simulink model "MPC_FOC"  (R2021a)
settings: Solver=VariableStepAuto  StartTime=0.0  StopTime=2  RelTol=1e-3
undefined symbols (not defined in the file): C1, JL, JM, K1, sigbuilder_block
libraries: powerlib_extras x9, spsDCVoltageSourceLib x4, spsPermanentMagnetSynchronousMachineLib x4, spsUniversalBridgeLib x4, spspowerguiLib x4, simulink x3, spsVoltageMeasurementLib x3, pid_lib x1
(part 1 of 2)
settings Model: Creator=86188  LastModifiedBy=86188

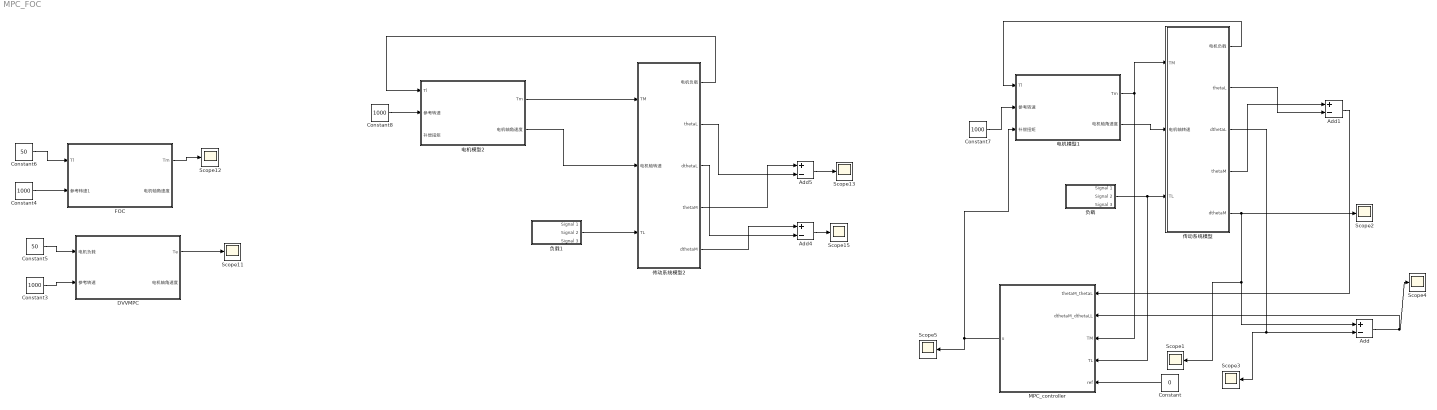
== system MPC_FOC ==
  Add{,1,4..5} (4 alike) : Sum  Inputs=+-
  Constant : Constant  Value=0
  Constant{3..4,7..8} (4 alike) : Constant  Value=1000
  Constant5 : Constant  Value=50
  Constant6 : Constant  Value=50
  DVVMPC : Subsystem
  FOC : Subsystem
  MPC_controller : MATLAB Function  TreatAsAtomicUnit=on
  Scope{1..5,11..13,15} (9 alike) : Scope
  传动系统模型 : Subsystem
  传动系统模型2 : Subsystem
  电机模型1 : Subsystem
  电机模型2 : Subsystem
  负载 : Subsystem  Tag=STV Subsys  LoadFcn=sigbuilder_block('load');  StartFcn=sigbuilder_block('start');  StopFcn=sigbuilder_block('stop');  ClipboardFcn=sigbuilder_block('clipboard');  mask(Sigbuilder block){tuvar=[0:10]}
      mask help: Simulink:masks:SigbuilderBlock_MD
      mask init:
      | if ~strcmp(get_param(bdroot(gcbh),'SimulationStatus'),'stopped') tuvar = sigbuilder_block('maskInit'); end
      settings: CopyFcn=sigbuilder_block('copy');  DeleteFcn=sigbuilder_block('delete');  ModelCloseFcn=sigbuilder_block('modelClose');  PreSaveFcn=sigbuilder_block('preSave');  PauseFcn=sigbuilder_block('pause');  ContinueFcn=sigbuilder_block('continue');  NameChangeFcn=sigbuilder_block('namechange');  OpenFcn=sigbuilder_block('open',[5.4 36 1141.2 517.8 ]);  CloseFcn=sigbuilder_block('close');
      mask Display: plot(0, 0, 100, 100,[2, 2, 32, 32, 2], [68, 8, 8, 68, 68],[32, 2], [38, 38], [32, 19, 2],[53, 60, 44], [32, 17, 17, 2],[16, 16, 31, 31]);txt = getActiveGroup(gcbh);text(2, 100, txt,'verticalAlignment', 'top');
  负载1 : Subsystem  Tag=STV Subsys  LoadFcn=sigbuilder_block('load');  StartFcn=sigbuilder_block('start');  StopFcn=sigbuilder_block('stop');  ClipboardFcn=sigbuilder_block('clipboard');  mask(Sigbuilder block){tuvar=[0:10]}
      mask help: Simulink:masks:SigbuilderBlock_MD
      mask init:
      | if ~strcmp(get_param(bdroot(gcbh),'SimulationStatus'),'stopped') tuvar = sigbuilder_block('maskInit'); end
      settings: CopyFcn=sigbuilder_block('copy');  DeleteFcn=sigbuilder_block('delete');  ModelCloseFcn=sigbuilder_block('modelClose');  PreSaveFcn=sigbuilder_block('preSave');  PauseFcn=sigbuilder_block('pause');  ContinueFcn=sigbuilder_block('continue');  NameChangeFcn=sigbuilder_block('namechange');  OpenFcn=sigbuilder_block('open',[5.4 36 1141.2 517.8 ]);  CloseFcn=sigbuilder_block('close');
      mask Display: plot(0, 0, 100, 100,[2, 2, 32, 32, 2], [68, 8, 8, 68, 68],[32, 2], [38, 38], [32, 19, 2],[53, 60, 44], [32, 17, 17, 2],[16, 16, 31, 31]);txt = getActiveGroup(gcbh);text(2, 100, txt,'verticalAlignment', 'top');
  wires:
  传动系统模型/1(电机负载) -> 电机模型1/1(Tl)
  传动系统模型/3(dthetaL) -> Scope3/1, Add/2
  负载/2(Signal 2) -> MPC_controller/4(TL), 传动系统模型/3(TL)
  Add/1 -> MPC_controller/2(dthetaM_dthetaLL), Scope4/1
  传动系统模型/5(dthetaM) -> Scope2/1, Add/1, Scope1/1
  电机模型1/2(电机轴角速度) -> 传动系统模型/2(电机轴转速)
  传动系统模型/2(thetaL) -> Add1/2
  传动系统模型/4(thetaM) -> Add1/1
  Add1/1 -> MPC_controller/1(thetaM_thetaL)
  Constant/1 -> MPC_controller/5(ref)
  MPC_controller/1(u) -> Scope5/1, 电机模型1/3(补偿扭矩)
  电机模型1/1(Tm) -> MPC_controller/3(TM), 传动系统模型/1(TM)
  Constant7/1 -> 电机模型1/2(参考转速)
  Constant3/1 -> DVVMPC/2(参考转速)
  Constant5/1 -> DVVMPC/1(电机负载)
  Constant6/1 -> FOC/1(Tl)
  DVVMPC/1(Te) -> Scope11/1
  FOC/1(Tm) -> Scope12/1
  传动系统模型2/4(thetaM) -> Add5/1
  传动系统模型2/1(电机负载) -> 电机模型2/1(Tl)
  电机模型2/2(电机轴角速度) -> 传动系统模型2/2(电机轴转速)
  传动系统模型2/2(thetaL) -> Add5/2
  电机模型2/1(Tm) -> 传动系统模型2/1(TM)
  Constant8/1 -> 电机模型2/2(参考转速)
  负载1/2(Signal 2) -> 传动系统模型2/3(TL)
  Constant4/1 -> FOC/2(参考转速1)
  Add5/1 -> Scope13/1
  Add4/1 -> Scope15/1
  传动系统模型2/5(dthetaM) -> Add4/1
  传动系统模型2/3(dthetaL) -> Add4/2

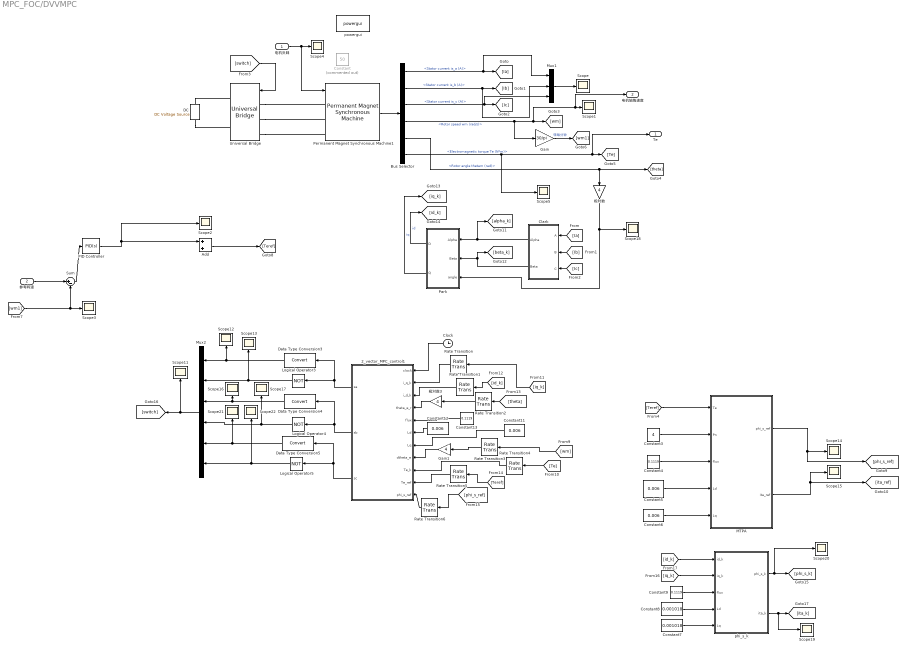
== system MPC_FOC/DVVMPC ==
  电机负载 : Inport
  参考转速 : Inport  Port=2
  2_vector_MPC_control1 : MATLAB Function  TreatAsAtomicUnit=on  SystemSampleTime=1e-5
  Add : Sum
  Bus Selector : BusSelector  OutputSignals=Stator current is_a (A),Stator current is_b (A),Stator current is_c (A),Rotor speed wm (rad/s),Rotor angle thetam (rad),Electromagnetic torque Te (N*m)
  Clark : Subsystem
  Clock : Clock
  Constant : Constant  Commented=on  Value=50
  Constant{5..6,11..12} (4 alike) : Constant  Value=0.006
  Constant13 : Constant  Value=0.1119
  Constant3 : Constant  Value=4
  Constant4 : Constant  Value=0.1119
  Constant7 : Constant  Value=0.001018
  Constant8 : Constant  Value=0.001018
  Constant9 : Constant  Value=0.1119
  DC : spsDCVoltageSourceLib/DC Voltage Source  Amplitude=400  Measurements=None
  Data Type Conversion3 : DataTypeConversion
  Data Type Conversion4 : DataTypeConversion
  Data Type Conversion5 : DataTypeConversion
  Gain : Gain  Gain=30/pi
  Gain1 : Gain  Gain=4
  Logical Operator3 : Logic  Operator=NOT  AllPortsSameDT=off  OutDataTypeStr=boolean
  Logical Operator4 : Logic  Operator=NOT  AllPortsSameDT=off  OutDataTypeStr=boolean
  Logical Operator5 : Logic  Operator=NOT  AllPortsSameDT=off  OutDataTypeStr=boolean
  MTPA : MATLAB Function  TreatAsAtomicUnit=on
  Mux1 : Mux  Inputs=3
  Mux2 : Mux  Inputs=6
  PID Controller : pid_lib/PID Controller  Controller=PID  Form=Parallel  TimeDomain=Continuous-time  UseExternalTs=off  SampleTime=-1  IntegratorMethod=Forward Euler  FilterMethod=Forward Euler  ControllerParametersSource=internal  P=2  I=0.125  D=0.01  UseFilter=on  N=100  TunerSelectOption=Transfer Function Based (PID Tuner App)  InitialConditionSource=internal  InitialConditionForIntegrator=0  InitialConditionForFilter=0  DifferentiatorICPrevScaledInput=0  ExternalReset=none  TrackingMode=off  Kt=1  LimitOutput=on  SatLimitsSource=internal  UpperSaturationLimit=140  LowerSaturationLimit=-200  LinearizeAsGain=on  AntiWindupMode=none  Kb=1  POutMin=[]  POutMax=[]  IOutMin=[]  IOutMax=[]  DOutMin=[]  DOutMax=[]  NOutMin=[]  NOutMax=[]  SumOutMin=[]  SumOutMax=[]  SaturationOutMin=[]  SaturationOutMax=[]  PParamMin=[]  PParamMax=[]  IParamMin=[]  IParamMax=[]  DParamMin=[]  DParamMax=[]  NParamMin=[]  NParamMax=[]  KbParamMin=[]  KbParamMax=[]  KtParamMin=[]  KtParamMax=[]  KbOutMin=[]  KbOutMax=[]  KtOutMin=[]  KtOutMax=[]  IntegratorOutMin=[]  IntegratorOutMax=[]  FilterOutMin=[]  FilterOutMax=[]  SumI1OutMin=[]  SumI1OutMax=[]  SumI2OutMin=[]  SumI2OutMax=[]  SumI3OutMin=[]  SumI3OutMax=[]  SumI4OutMin=[]  SumI4OutMax=[]  SumDOutMin=[]  SumDOutMax=[]  DifferentiatorOutMin=[]  DifferentiatorOutMax=[]  FilterDiffOutCoefMin=[]  FilterDiffOutCoefMax=[]  ReciprocalOutMin=[]  ReciprocalOutMax=[]  SumDenOutMin=[]  SumDenOutMax=[]  SumNumOutMin=[]  SumNumOutMax=[]  DivideOutMin=[]  DivideOutMax=[]  UdiffTsProdOutMin=[]  UdiffTsProdOutMax=[]  NTsProdOutMin=[]  NTsProdOutMax=[]  UintegralTsProdOutMin=[]  UintegralTsProdOutMax=[]  UngainTsProdOutMin=[]  UngainTsProdOutMax=[]  IntegratorContinuousStateAttributes=''  IntegratorStateMustResolveToSignalObject=off  IntegratorRTWStateStorageClass=Auto  FilterContinuousStateAttributes=''  FilterStateMustResolveToSignalObject=off  FilterRTWStateStorageClass=Auto  ParallelPVariant=InternalParameters  IdealPVariant=Disabled  IVariant=InternalParameters  DVariant=InternalParameters  IntegratorVariant=Continuous  SatVariant=Enabled  AWVariant=Passthrough  PCopyVariant=Disabled  TRVariant=Disabled  FdbkBlocksVariant=Forward  IdealPFdbkVariant=Disabled  SatFdbkVariant=Disabled  DerivativeFilterVariant=ContFilter  NVariant=InternalParameters  NCopyVariant=Disabled  FilterICVariant=InternalICsFilter  IntegratorICVariant=InternalICs  ExternalResetVariant=Disabled  TRSumVariant=Passthrough  SumFdbkVariant=Disabled  SumVariant=Sum_PID  TsampFilterVariant=InternalTs  TsampNgainVariant=Passthrough  TsampIntegralVariant=Passthrough  ExternalSaturationOutDataTypeStr=Inherit: Same as second input
  Park : Subsystem
  Permanent Magnet Synchronous Machine1 : spsPermanentMagnetSynchronousMachineLib/Permanent Magnet Synchronous Machine  NbPhases=3  FluxDistribution=Sinusoidal  RotorType=Salient-pole  MechanicalLoad=Torque Tm  PresetModel=No  ShowDetailedParameters=on  MeasurementBus=off  Resistance=0.11  Inductance=8.5e-3  dqInductances=[0.006 0.006]  La=0.000835  MachineConstant=Flux linkage established by magnets (V.s)  Flux=0.1119  VoltageCst=81.1857  TorqueCst=0.6714  Flat=120  Mechanical=[0.04 0.0002024 4 0]  PolePairs=4  InitialConditions=[0,0, 0,0]  InitialConditions5ph=[0 0 0 0 0 0]  RefAngle=Aligned with phase A axis (original Park)  IterativeDiscreteModel=Trapezoidal non iterative  TsBlock=-1  TsPowergui=0
  Rate Transition{,1..6} (7 alike) : RateTransition  OutPortSampleTime=1e-4
  Scope{,1..5,11..22} (18 alike) : Scope
  Sum : Sum  Inputs=|+-
  Universal Bridge : spsUniversalBridgeLib/Universal Bridge  Arms=3  SnubberResistance=1e5  SnubberCapacitance=inf  Device=IGBT / Diodes  Ron=1e-3  Lon=0  ForwardVoltages="[  0  0  ]"  ForwardVoltage=0  GTOparameters=[ 10e-6 , 20e-6 ]  IGBTparameters=[ 1e-6 , 2e-6 ]  Measurements=None  Measurements_2=None  converterType=Rectifier
  phi_s_k : MATLAB Function  TreatAsAtomicUnit=on
  powergui : spspowerguiLib/powergui  Priority=1  SimulationMode=Discrete  SampleTime=1e-6  frequency=60  Iterations=50  frequencyindice=0  Pbase=100e6  ErrMax=1e-4  UnitsV=kV  UnitsW=MW  buscounter=0  FunctionMessages=off  echomessages=off  EnableUseOfTLC=off  CurrentSourceSwitches=off  DisableSnubberDevices=off  DisableRonSwitches=off  DisableVfSwitches=off  DisplayEquations=off  AutomaticDiscreteSolvers=off  SolverType=Tustin/Backward Euler (TBE)  Interpol=off  ExternalGateDelay=off  methode=off  Ts=100  x0status=blocks  SPID=on  SwTol=0  HookPort=off  NonlinearTolerance=1e-4  nMaxIteration=100  ContinueOnMaxIteration=off  RestoreLinks=warning  ResistiveCurrentMeasurement=off  Frange=[0:2:500]  Ylog=off  Xlog=on  ShowGrid=off  save=off  variable=ZData  structure=0  ZoomFFT=off  StartTime=0.0  cycles=1  DisplayStyle=1  fundamental=60  FreqAxis=off  MaxFrequency=1000  frequencyindicesteady=1  RmsSteady=1  display=off
  极对数 : Gain  Gain=4
  极对数3 : Gain  Gain=4
  Te : Outport
  电机轴角速度 : Outport  Port=2
  wires:
  参考转速/1 -> Sum/1
  Add/1 -> [Teref]
  电机负载/1 -> Scope4/1, Permanent Magnet Synchronous Machine1/1
  Rate Transition6/1 -> 2_vector_MPC_control1/11(phi_s_ref)
  Rate Transition5/1 -> 2_vector_MPC_control1/10(Te_ref)
  Rate Transition4/1 -> 2_vector_MPC_control1/9(Te_k)
  Rate Transition3/1 -> Gain1/1
  Rate Transition2/1 -> 极对数3/1
  Rate Transition1/1 -> 2_vector_MPC_control1/3(i_d_k)
  Rate Transition/1 -> 2_vector_MPC_control1/2(i_q_k)
  phi_s_k/2(ita_k) -> [ita_k], Scope19/1
  极对数3/1 -> 2_vector_MPC_control1/4(theta_e_r)
  Mux2/1 -> [switch], Scope11/1
  Logical Operator5/1 -> Scope22/1, Mux2/6
  Data Type Conversion5/1 -> Scope21/1, Mux2/5
  Logical Operator4/1 -> Scope17/1, Mux2/4
  Data Type Conversion4/1 -> Scope16/1, Mux2/3
  Logical Operator3/1 -> Scope13/1, Mux2/2
  Data Type Conversion3/1 -> Scope12/1, Mux2/1
  2_vector_MPC_control1/3(sc) -> Logical Operator5/1, Data Type Conversion5/1
  2_vector_MPC_control1/2(sb) -> Logical Operator4/1, Data Type Conversion4/1
  2_vector_MPC_control1/1(sa) -> Logical Operator3/1, Data Type Conversion3/1
  [id_k] -> phi_s_k/1(id_k)
  [iq_k] -> phi_s_k/2(iq_k)
  phi_s_k/1(phi_s_k) -> Scope20/1, [phi_s_k]
  Constant9/1 -> phi_s_k/3(flux)
  Constant8/1 -> phi_s_k/4(Ld)
  Constant7/1 -> phi_s_k/5(Lq)
  MTPA/1(phi_s_ref) -> Scope14/1, [phi_s_ref]
  MTPA/2(ita_ref) -> [ita_ref], Scope15/1
  Constant6/1 -> MTPA/5(Lq)
  Constant5/1 -> MTPA/4(Ld)
  Constant4/1 -> MTPA/3(flux)
  Constant3/1 -> MTPA/2(Pn)
  [Teref] -> MTPA/1(Te)
  Clock/1 -> 2_vector_MPC_control1/1(clock)
  Permanent Magnet Synchronous Machine1/1 -> Bus Selector/1
  Bus Selector/1 -> Mux1/1, [Ia]  "<Stator current is_a (A)>"
  Bus Selector/2 -> Mux1/2, [Ib]  "<Stator current is_b (A)>"
  Bus Selector/3 -> Mux1/3, [Ic]  "<Stator current is_c (A)>"
  Bus Selector/4 -> Gain/1, Scope1/1, 电机轴角速度/1, [wm]  "<Rotor speed wm (rad/s)>"
  Bus Selector/5 -> 极对数/1, [theta]  "<Rotor angle thetam (rad)>"
  Bus Selector/6 -> [Te], Te/1, Scope5/1  "<Electromagnetic torque Te (N*m)>"
  Gain/1 -> [wm1]  "转每分钟"
  Clark/1(Alpha) -> Park/1(Alpha), [alpha_k]
  Clark/2(Beta) -> Park/2(Beta), [beta_k]
  [Ia] -> Clark/1(A)
  [Ib] -> Clark/2(B)
  [Ic] -> Clark/3(C)
  极对数/1 -> Park/3(angle), Scope18/1
  Park/1(D) -> [id_k]  "id"
  Park/2(Q) -> [iq_k]  "iq"
  [switch] -> Universal Bridge/1
  Mux1/1 -> Scope/1
  Sum/1 -> PID Controller/1
  [wm1] -> Scope3/1, Sum/2
  PID Controller/1 -> Scope2/1, Add/1
  Gain1/1 -> 2_vector_MPC_control1/8(dtheta_e)
  Constant12/1 -> 2_vector_MPC_control1/6(Ld)
  Constant11/1 -> 2_vector_MPC_control1/7(Lq)
  Constant13/1 -> 2_vector_MPC_control1/5(flux)
  [Teref] -> Rate Transition5/1
  [phi_s_ref] -> Rate Transition6/1
  [iq_k] -> Rate Transition/1
  [id_k] -> Rate Transition1/1
  [theta] -> Rate Transition2/1
  [wm] -> Rate Transition3/1
  [Te] -> Rate Transition4/1
  connections:
  Universal Bridge/LConn2 -- Permanent Magnet Synchronous Machine1/LConn2
  Universal Bridge/LConn3 -- Permanent Magnet Synchronous Machine1/LConn3
  Universal Bridge/LConn1 -- Permanent Magnet Synchronous Machine1/LConn1
  DC/RConn1 -- Universal Bridge/RConn1
  DC/LConn1 -- Universal Bridge/RConn2

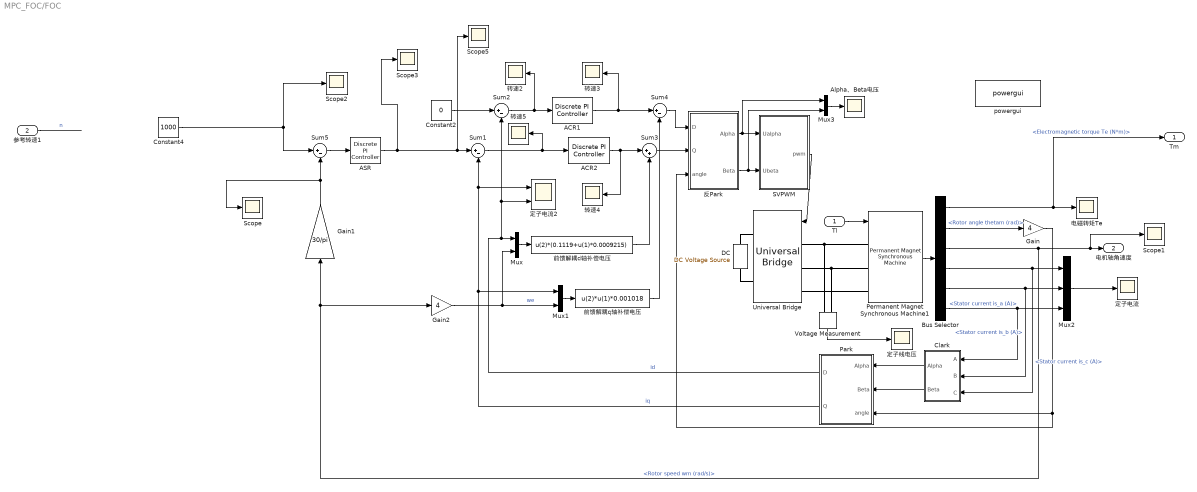
== system MPC_FOC/FOC ==
  Tl : Inport
  参考转速1 : Inport  Port=2
  ACR1 : powerlib_extras/Discrete  Control Blocks/Discrete PI Controller  Kp=4  Ki=80  Par_Limits=[560*0.9*sqrt(1/3) -560*0.9*sqrt(1/3)]  Init=0  Ts=1e-6
  ACR2 : powerlib_extras/Discrete  Control Blocks/Discrete PI Controller  Kp=4  Ki=80  Par_Limits=[560*0.9*sqrt(1/3) -560*0.9*sqrt(1/3)]  Init=0  Ts=1e-6
  ASR : powerlib_extras/Discrete  Control Blocks/Discrete PI Controller  Kp=5  Ki=200  Par_Limits=[200 -200]  Init=0  Ts=1e-6
  Alpha、Beta电压 : Scope
  Bus Selector : BusSelector  OutputSignals=Electromagnetic torque Te (N*m),Rotor angle thetam (rad),Rotor speed wm (rad/s),Stator current is_c (A),Stator current is_b (A),Stator current is_a (A)
  Clark : Subsystem
  Constant2 : Constant  Value=0
  Constant4 : Constant  Value=1000
  DC : spsDCVoltageSourceLib/DC Voltage Source  Amplitude=560  Measurements=None
  Gain : Gain  Gain=4
  Gain1 : Gain  Gain=30/pi
  Gain2 : Gain  Gain=4
  Mux : Mux  Inputs=2
  Mux1 : Mux  Inputs=2
  Mux2 : Mux  Inputs=3
  Mux3 : Mux  Inputs=2
  Park : Subsystem
  Permanent Magnet Synchronous Machine1 : spsPermanentMagnetSynchronousMachineLib/Permanent Magnet Synchronous Machine  NbPhases=3  FluxDistribution=Sinusoidal  RotorType=Salient-pole  MechanicalLoad=Torque Tm  PresetModel=No  ShowDetailedParameters=on  MeasurementBus=off  Resistance=0.11  Inductance=8.5e-3  dqInductances=[0.0009215 0.001018]  La=0.000835  MachineConstant=Flux linkage established by magnets (V.s)  Flux=0.1119  VoltageCst=81.1857  TorqueCst=0.6714  Flat=120  Mechanical=[0.04 0.0002024 4 0]  PolePairs=4  InitialConditions=[0,0, 0,0]  InitialConditions5ph=[0 0 0 0 0 0]  RefAngle=Aligned with phase A axis (original Park)  IterativeDiscreteModel=Trapezoidal non iterative  TsBlock=-1  TsPowergui=0
  SVPWM : Subsystem
  Scope{,1..3,5} (5 alike) : Scope
  Sum{1..2,4..5} (4 alike) : Sum  Inputs=|+-
  Sum3 : Sum  Inputs=|++
  Universal Bridge : spsUniversalBridgeLib/Universal Bridge  Arms=3  SnubberResistance=1e5  SnubberCapacitance=inf  Device=IGBT / Diodes  Ron=1e-3  Lon=0  ForwardVoltages="[  0  0  ]"  ForwardVoltage=0  GTOparameters=[ 10e-6 , 20e-6 ]  IGBTparameters=[ 1e-6 , 2e-6 ]  Measurements=None  Measurements_2=None  converterType=Rectifier
  Voltage Measurement : spsVoltageMeasurementLib/Voltage Measurement  PhasorSimulation=off  OutputType=Complex  PSBequivalent=0
  powergui : spspowerguiLib/powergui  Priority=1  SimulationMode=Discrete  SampleTime=1e-5  frequency=60  Iterations=50  frequencyindice=0  Pbase=100e6  ErrMax=1e-4  UnitsV=kV  UnitsW=MW  buscounter=0  FunctionMessages=off  echomessages=off  EnableUseOfTLC=off  CurrentSourceSwitches=off  DisableSnubberDevices=off  DisableRonSwitches=off  DisableVfSwitches=off  DisplayEquations=off  AutomaticDiscreteSolvers=off  SolverType=Tustin  Interpol=off  ExternalGateDelay=off  methode=off  Ts=0  x0status=blocks  SPID=off  SwTol=0  HookPort=off  NonlinearTolerance=1e-4  nMaxIteration=100  ContinueOnMaxIteration=off  RestoreLinks=warning  ResistiveCurrentMeasurement=off  Frange=[0:2:500]  Ylog=off  Xlog=on  ShowGrid=off  save=off  variable=ZData  structure=ScopeData7  ZoomFFT=on  StartTime=2.5  cycles=3  DisplayStyle=1  fundamental=60  FreqAxis=off  MaxFrequency=2000  frequencyindicesteady=1  RmsSteady=1  display=off
  前馈解耦d轴补偿电压 : Fcn  Expr=u(2)*(0.1119+u(1)*0.0009215)
  前馈解耦q轴补偿电压 : Fcn  Expr=u(2)*u(1)*0.001018
  反Park : Subsystem
  定子电流 : Scope
  定子电流2 : Scope  NumInputPorts=2
  定子线电压 : Scope
  电磁转矩Te : Scope
  转速{2..5} (4 alike) : Scope
  Tm : Outport
  电机轴角速度 : Outport  Port=2
  wires:
  ASR/1 -> Sum1/1, Scope5/1, Scope3/1
  Constant4/1 -> Scope2/1, Sum5/1
  Gain1/1 -> Scope/1, Sum5/2
  Tl/1 -> Permanent Magnet Synchronous Machine1/1
  Voltage Measurement/1 -> 定子线电压/1
  前馈解耦q轴补偿电压/1 -> Sum4/2
  Sum2/1 -> ACR1/1, 转速2/1
  Mux2/1 -> 定子电流/1
  Bus Selector/6 -> Clark/1(A), Mux2/3  "<Stator current is_a (A)>"
  Sum5/1 -> ASR/1
  Clark/1(Alpha) -> Park/1(Alpha)
  Permanent Magnet Synchronous Machine1/1 -> Bus Selector/1
  Park/2(Q) -> Sum1/2, 定子电流2/1, Mux1/1  "iq"
  Clark/2(Beta) -> Park/2(Beta)
  Sum1/1 -> ACR2/1, 转速5/1
  Mux3/1 -> Alpha、Beta电压/1
  反Park/1(Alpha) -> SVPWM/1(Ualpha), Mux3/1
  Bus Selector/3 -> 电机轴角速度/1, Scope1/1, Gain1/1, Gain2/1  "<Rotor speed wm (rad/s)>"
  Mux/1 -> 前馈解耦d轴补偿电压/1
  反Park/2(Beta) -> SVPWM/2(Ubeta), Mux3/2
  Sum3/1 -> 反Park/2(Q)
  Park/1(D) -> Mux/1, Sum2/2, 定子电流2/2  "id"
  Bus Selector/1 -> 电磁转矩Te/1, Tm/1  "<Electromagnetic torque Te (N*m)>"
  Bus Selector/5 -> Clark/2(B), Mux2/2  "<Stator current is_b (A)>"
  Bus Selector/2 -> Gain/1  "<Rotor angle thetam (rad)>"
  前馈解耦d轴补偿电压/1 -> Sum3/2
  ACR2/1 -> Sum3/1, 转速4/1
  Sum4/1 -> 反Park/1(D)
  SVPWM/1(pwm) -> Universal Bridge/1
  Mux1/1 -> 前馈解耦q轴补偿电压/1
  Gain2/1 -> Mux/2, Mux1/2  "we"
  Gain/1 -> Park/3(angle), 反Park/3(angle)
  Constant2/1 -> Sum2/1
  Bus Selector/4 -> Clark/3(C), Mux2/1  "<Stator current is_c (A)>"
  ACR1/1 -> Sum4/1, 转速3/1
  参考转速1/1 -> ?  "n"
  connections:
  Voltage Measurement/LConn1 -- Permanent Magnet Synchronous Machine1/LConn1 -- Universal Bridge/LConn1
  Voltage Measurement/LConn2 -- Permanent Magnet Synchronous Machine1/LConn2 -- Universal Bridge/LConn2
  DC/RConn1 -- Universal Bridge/RConn1
  Permanent Magnet Synchronous Machine1/LConn3 -- Universal Bridge/LConn3
  DC/LConn1 -- Universal Bridge/RConn2

== system MPC_FOC/传动系统模型 ==
  TM : Inport
  电机轴转速 : Inport  Port=2
  TL : Inport  Port=3
  Fcn1 : Subsystem
  Fcn2 : Subsystem
  电机负载 : Outport
  thetaL : Outport  Port=2
  dthetaL : Outport  Port=3
  thetaM : Outport  Port=4
  dthetaM : Outport  Port=5
  wires:
  Fcn2/1(d2thetaL) -> Fcn1/2(d2theta1)
  TM/1 -> Fcn1/1(TM)
  电机轴转速/1 -> Fcn1/3(电机轴转速)
  Fcn1/1(d2theta) -> Fcn2/2(d2thata)
  Fcn1/2(电机负载) -> 电机负载/1
  Fcn1/3(thetaM) -> thetaM/1
  Fcn1/4(dthetaM) -> dthetaM/1
  TL/1 -> Fcn2/1(TL)
  Fcn2/2(thetaL) -> thetaL/1
  Fcn2/3(dthetaL) -> dthetaL/1

== system MPC_FOC/传动系统模型2 ==
  TM : Inport
  电机轴转速 : Inport  Port=2
  TL : Inport  Port=3
  Fcn1 : Subsystem
  Fcn2 : Subsystem
  电机负载 : Outport
  thetaL : Outport  Port=2
  dthetaL : Outport  Port=3
  thetaM : Outport  Port=4
  dthetaM : Outport  Port=5
  wires:
  Fcn2/3(dthetaL) -> dthetaL/1
  Fcn2/2(thetaL) -> thetaL/1
  TL/1 -> Fcn2/1(TL)
  Fcn1/4(dthetaM) -> dthetaM/1
  Fcn1/3(thetaM) -> thetaM/1
  Fcn1/2(电机负载) -> 电机负载/1
  Fcn1/1(d2theta) -> Fcn2/2(d2thata)
  电机轴转速/1 -> Fcn1/3(电机轴转速)
  TM/1 -> Fcn1/1(TM)
  Fcn2/1(d2thetaL) -> Fcn1/2(d2theta1)

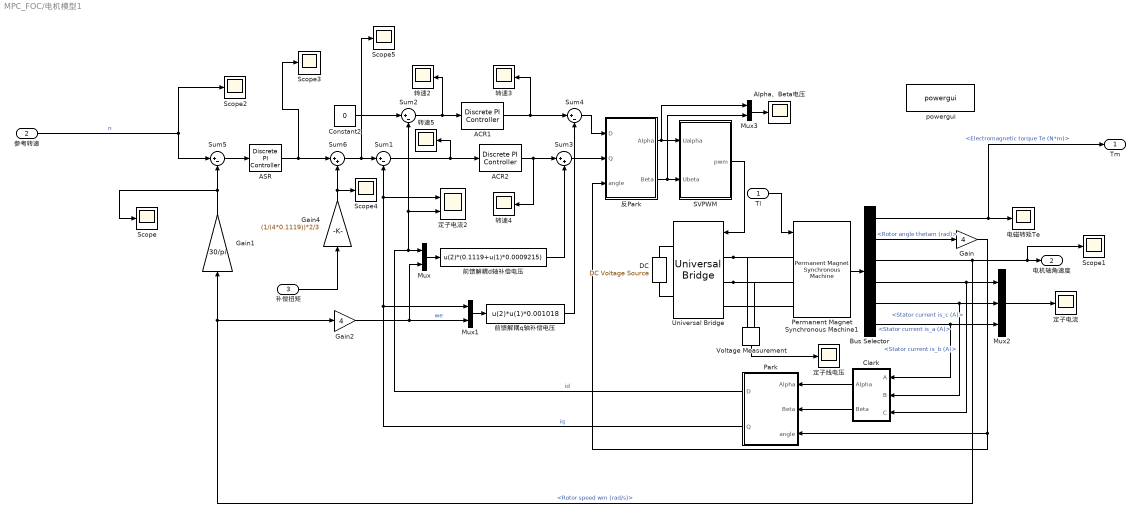
== system MPC_FOC/电机模型1 ==
  Tl : Inport
  参考转速 : Inport  Port=2
  补偿扭矩 : Inport  Port=3
  ACR1 : powerlib_extras/Discrete  Control Blocks/Discrete PI Controller  Kp=4  Ki=80  Par_Limits=[560*0.9*sqrt(1/3) -560*0.9*sqrt(1/3)]  Init=0  Ts=1e-6
  ACR2 : powerlib_extras/Discrete  Control Blocks/Discrete PI Controller  Kp=4  Ki=80  Par_Limits=[560*0.9*sqrt(1/3) -560*0.9*sqrt(1/3)]  Init=0  Ts=1e-6
  ASR : powerlib_extras/Discrete  Control Blocks/Discrete PI Controller  Kp=5  Ki=200  Par_Limits=[200 -200]  Init=0  Ts=-1
  Alpha、Beta电压 : Scope
  Bus Selector : BusSelector  OutputSignals=Electromagnetic torque Te (N*m),Rotor angle thetam (rad),Rotor speed wm (rad/s),Stator current is_c (A),Stator current is_b (A),Stator current is_a (A)
  Clark : Subsystem
  Constant2 : Constant  Value=0
  DC : spsDCVoltageSourceLib/DC Voltage Source  Amplitude=560  Measurements=None
  Gain : Gain  Gain=4
  Gain1 : Gain  Gain=30/pi
  Gain2 : Gain  Gain=4
  Gain4 : Gain  Gain=(1/(4*0.1119))*2/3
  Mux : Mux  Inputs=2
  Mux1 : Mux  Inputs=2
  Mux2 : Mux  Inputs=3
  Mux3 : Mux  Inputs=2
  Park : Subsystem
  Permanent Magnet Synchronous Machine1 : spsPermanentMagnetSynchronousMachineLib/Permanent Magnet Synchronous Machine  NbPhases=3  FluxDistribution=Sinusoidal  RotorType=Salient-pole  MechanicalLoad=Torque Tm  PresetModel=No  ShowDetailedParameters=on  MeasurementBus=off  Resistance=0.11  Inductance=8.5e-3  dqInductances=[0.0009215 0.001018]  La=0.000835  MachineConstant=Flux linkage established by magnets (V.s)  Flux=0.1119  VoltageCst=81.1857  TorqueCst=0.6714  Flat=120  Mechanical=[0.04 0.0002024 4 0]  PolePairs=4  InitialConditions=[0,0, 0,0]  InitialConditions5ph=[0 0 0 0 0 0]  RefAngle=Aligned with phase A axis (original Park)  IterativeDiscreteModel=Trapezoidal non iterative  TsBlock=-1  TsPowergui=0
  SVPWM : Subsystem
  Scope{,1..5} (6 alike) : Scope
  Sum{1..2,4..5} (4 alike) : Sum  Inputs=|+-
  Sum3 : Sum  Inputs=|++
  Sum6 : Sum  Inputs=|++
  Universal Bridge : spsUniversalBridgeLib/Universal Bridge  Arms=3  SnubberResistance=1e5  SnubberCapacitance=inf  Device=IGBT / Diodes  Ron=1e-3  Lon=0  ForwardVoltages="[  0  0  ]"  ForwardVoltage=0  GTOparameters=[ 10e-6 , 20e-6 ]  IGBTparameters=[ 1e-6 , 2e-6 ]  Measurements=None  Measurements_2=None  converterType=Rectifier
  Voltage Measurement : spsVoltageMeasurementLib/Voltage Measurement  PhasorSimulation=off  OutputType=Complex  PSBequivalent=0
  powergui : spspowerguiLib/powergui  Priority=1  SimulationMode=Discrete  SampleTime=1e-5  frequency=60  Iterations=50  frequencyindice=0  Pbase=100e6  ErrMax=1e-4  UnitsV=kV  UnitsW=MW  buscounter=0  FunctionMessages=off  echomessages=off  EnableUseOfTLC=off  CurrentSourceSwitches=off  DisableSnubberDevices=off  DisableRonSwitches=off  DisableVfSwitches=off  DisplayEquations=off  AutomaticDiscreteSolvers=off  SolverType=Tustin  Interpol=off  ExternalGateDelay=off  methode=off  Ts=0  x0status=blocks  SPID=off  SwTol=0  HookPort=off  NonlinearTolerance=1e-4  nMaxIteration=100  ContinueOnMaxIteration=off  RestoreLinks=warning  ResistiveCurrentMeasurement=off  Frange=[0:2:500]  Ylog=off  Xlog=on  ShowGrid=off  save=off  variable=ZData  structure=ScopeData7  ZoomFFT=on  StartTime=2.5  cycles=3  DisplayStyle=1  fundamental=60  FreqAxis=off  MaxFrequency=2000  frequencyindicesteady=1  RmsSteady=1  display=off
  前馈解耦d轴补偿电压 : Fcn  Expr=u(2)*(0.1119+u(1)*0.0009215)
  前馈解耦q轴补偿电压 : Fcn  Expr=u(2)*u(1)*0.001018
  反Park : Subsystem
  定子电流 : Scope
  定子电流2 : Scope  NumInputPorts=2
  定子线电压 : Scope
  电磁转矩Te : Scope
  转速{2..5} (4 alike) : Scope
  Tm : Outport
  电机轴角速度 : Outport  Port=2
  wires:
  ACR1/1 -> 转速3/1, Sum4/1
  Bus Selector/4 -> Mux2/1, Clark/3(C)  "<Stator current is_c (A)>"
  Constant2/1 -> Sum2/1
  Gain/1 -> 反Park/3(angle), Park/3(angle)
  Gain2/1 -> Mux1/2, Mux/2  "we"
  Mux1/1 -> 前馈解耦q轴补偿电压/1
  SVPWM/1(pwm) -> Universal Bridge/1
  Sum4/1 -> 反Park/1(D)
  ACR2/1 -> 转速4/1, Sum3/1
  前馈解耦d轴补偿电压/1 -> Sum3/2
  参考转速/1 -> Sum5/1, Scope2/1  "n"
  Bus Selector/2 -> Gain/1  "<Rotor angle thetam (rad)>"
  Bus Selector/5 -> Mux2/2, Clark/2(B)  "<Stator current is_b (A)>"
  Bus Selector/1 -> Tm/1, 电磁转矩Te/1  "<Electromagnetic torque Te (N*m)>"
  Park/1(D) -> 定子电流2/2, Sum2/2, Mux/1  "id"
  Sum3/1 -> 反Park/2(Q)
  反Park/2(Beta) -> Mux3/2, SVPWM/2(Ubeta)
  Mux/1 -> 前馈解耦d轴补偿电压/1
  Bus Selector/3 -> Gain2/1, Gain1/1, Scope1/1, 电机轴角速度/1  "<Rotor speed wm (rad/s)>"
  反Park/1(Alpha) -> Mux3/1, SVPWM/1(Ualpha)
  Mux3/1 -> Alpha、Beta电压/1
  Sum1/1 -> 转速5/1, ACR2/1
  Clark/2(Beta) -> Park/2(Beta)
  Park/2(Q) -> Mux1/1, 定子电流2/1, Sum1/2  "iq"
  Permanent Magnet Synchronous Machine1/1 -> Bus Selector/1
  Clark/1(Alpha) -> Park/1(Alpha)
  Sum5/1 -> ASR/1
  Bus Selector/6 -> Mux2/3, Clark/1(A)  "<Stator current is_a (A)>"
  Mux2/1 -> 定子电流/1
  Sum2/1 -> 转速2/1, ACR1/1
  前馈解耦q轴补偿电压/1 -> Sum4/2
  Voltage Measurement/1 -> 定子线电压/1
  Tl/1 -> Permanent Magnet Synchronous Machine1/1
  Gain1/1 -> Sum5/2, Scope/1
  ASR/1 -> Scope3/1, Sum6/1
  Sum6/1 -> Scope5/1, Sum1/1
  补偿扭矩/1 -> Gain4/1
  Gain4/1 -> Scope4/1, Sum6/2
  connections:
  DC/LConn1 -- Universal Bridge/RConn2
  Permanent Magnet Synchronous Machine1/LConn3 -- Universal Bridge/LConn3
  DC/RConn1 -- Universal Bridge/RConn1
  Universal Bridge/LConn2 -- Permanent Magnet Synchronous Machine1/LConn2 -- Voltage Measurement/LConn2
  Universal Bridge/LConn1 -- Permanent Magnet Synchronous Machine1/LConn1 -- Voltage Measurement/LConn1

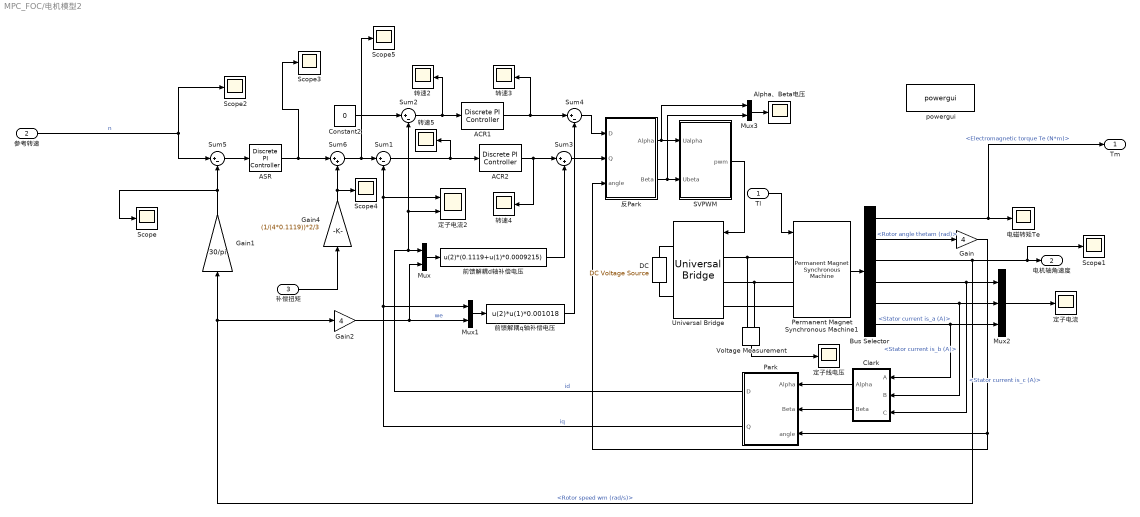
== system MPC_FOC/电机模型2 ==
  Tl : Inport
  参考转速 : Inport  Port=2
  补偿扭矩 : Inport  Port=3
  ACR1 : powerlib_extras/Discrete  Control Blocks/Discrete PI Controller  Kp=4  Ki=80  Par_Limits=[560*0.9*sqrt(1/3) -560*0.9*sqrt(1/3)]  Init=0  Ts=1e-6
  ACR2 : powerlib_extras/Discrete  Control Blocks/Discrete PI Controller  Kp=4  Ki=80  Par_Limits=[560*0.9*sqrt(1/3) -560*0.9*sqrt(1/3)]  Init=0  Ts=1e-6
  ASR : powerlib_extras/Discrete  Control Blocks/Discrete PI Controller  Kp=5  Ki=200  Par_Limits=[200 -200]  Init=0  Ts=-1
  Alpha、Beta电压 : Scope
  Bus Selector : BusSelector  OutputSignals=Electromagnetic torque Te (N*m),Rotor angle thetam (rad),Rotor speed wm (rad/s),Stator current is_c (A),Stator current is_b (A),Stator current is_a (A)
  Clark : Subsystem
  Constant2 : Constant  Value=0
  DC : spsDCVoltageSourceLib/DC Voltage Source  Amplitude=560  Measurements=None
  Gain : Gain  Gain=4
  Gain1 : Gain  Gain=30/pi
  Gain2 : Gain  Gain=4
  Gain4 : Gain  Gain=(1/(4*0.1119))*2/3
  Mux : Mux  Inputs=2
  Mux1 : Mux  Inputs=2
  Mux2 : Mux  Inputs=3
  Mux3 : Mux  Inputs=2
  Park : Subsystem
  Permanent Magnet Synchronous Machine1 : spsPermanentMagnetSynchronousMachineLib/Permanent Magnet Synchronous Machine  NbPhases=3  FluxDistribution=Sinusoidal  RotorType=Salient-pole  MechanicalLoad=Torque Tm  PresetModel=No  ShowDetailedParameters=on  MeasurementBus=off  Resistance=0.11  Inductance=8.5e-3  dqInductances=[0.0009215 0.001018]  La=0.000835  MachineConstant=Flux linkage established by magnets (V.s)  Flux=0.1119  VoltageCst=81.1857  TorqueCst=0.6714  Flat=120  Mechanical=[0.04 0.0002024 4 0]  PolePairs=4  InitialConditions=[0,0, 0,0]  InitialConditions5ph=[0 0 0 0 0 0]  RefAngle=Aligned with phase A axis (original Park)  IterativeDiscreteModel=Trapezoidal non iterative  TsBlock=-1  TsPowergui=0
  SVPWM : Subsystem
  Scope{,1..5} (6 alike) : Scope
  Sum{1..2,4..5} (4 alike) : Sum  Inputs=|+-
  Sum3 : Sum  Inputs=|++
  Sum6 : Sum  Inputs=|++
  Universal Bridge : spsUniversalBridgeLib/Universal Bridge  Arms=3  SnubberResistance=1e5  SnubberCapacitance=inf  Device=IGBT / Diodes  Ron=1e-3  Lon=0  ForwardVoltages="[  0  0  ]"  ForwardVoltage=0  GTOparameters=[ 10e-6 , 20e-6 ]  IGBTparameters=[ 1e-6 , 2e-6 ]  Measurements=None  Measurements_2=None  converterType=Rectifier
  Voltage Measurement : spsVoltageMeasurementLib/Voltage Measurement  PhasorSimulation=off  OutputType=Complex  PSBequivalent=0
  powergui : spspowerguiLib/powergui  Priority=1  SimulationMode=Discrete  SampleTime=1e-5  frequency=60  Iterations=50  frequencyindice=0  Pbase=100e6  ErrMax=1e-4  UnitsV=kV  UnitsW=MW  buscounter=0  FunctionMessages=off  echomessages=off  EnableUseOfTLC=off  CurrentSourceSwitches=off  DisableSnubberDevices=off  DisableRonSwitches=off  DisableVfSwitches=off  DisplayEquations=off  AutomaticDiscreteSolvers=off  SolverType=Tustin  Interpol=off  ExternalGateDelay=off  methode=off  Ts=0  x0status=blocks  SPID=off  SwTol=0  HookPort=off  NonlinearTolerance=1e-4  nMaxIteration=100  ContinueOnMaxIteration=off  RestoreLinks=warning  ResistiveCurrentMeasurement=off  Frange=[0:2:500]  Ylog=off  Xlog=on  ShowGrid=off  save=off  variable=ZData  structure=ScopeData7  ZoomFFT=on  StartTime=2.5  cycles=3  DisplayStyle=1  fundamental=60  FreqAxis=off  MaxFrequency=2000  frequencyindicesteady=1  RmsSteady=1  display=off
  前馈解耦d轴补偿电压 : Fcn  Expr=u(2)*(0.1119+u(1)*0.0009215)
  前馈解耦q轴补偿电压 : Fcn  Expr=u(2)*u(1)*0.001018
  反Park : Subsystem
  定子电流 : Scope
  定子电流2 : Scope  NumInputPorts=2
  定子线电压 : Scope
  电磁转矩Te : Scope
  转速{2..5} (4 alike) : Scope
  Tm : Outport
  电机轴角速度 : Outport  Port=2
  wires:
  Gain4/1 -> Sum6/2, Scope4/1
  补偿扭矩/1 -> Gain4/1
  Sum6/1 -> Sum1/1, Scope5/1
  ASR/1 -> Sum6/1, Scope3/1
  Gain1/1 -> Scope/1, Sum5/2
  Tl/1 -> Permanent Magnet Synchronous Machine1/1
  Voltage Measurement/1 -> 定子线电压/1
  前馈解耦q轴补偿电压/1 -> Sum4/2
  Sum2/1 -> ACR1/1, 转速2/1
  Mux2/1 -> 定子电流/1
  Bus Selector/6 -> Clark/1(A), Mux2/3  "<Stator current is_a (A)>"
  Sum5/1 -> ASR/1
  Clark/1(Alpha) -> Park/1(Alpha)
  Permanent Magnet Synchronous Machine1/1 -> Bus Selector/1
  Park/2(Q) -> Sum1/2, 定子电流2/1, Mux1/1  "iq"
  Clark/2(Beta) -> Park/2(Beta)
  Sum1/1 -> ACR2/1, 转速5/1
  Mux3/1 -> Alpha、Beta电压/1
  反Park/1(Alpha) -> SVPWM/1(Ualpha), Mux3/1
  Bus Selector/3 -> 电机轴角速度/1, Scope1/1, Gain1/1, Gain2/1  "<Rotor speed wm (rad/s)>"
  Mux/1 -> 前馈解耦d轴补偿电压/1
  反Park/2(Beta) -> SVPWM/2(Ubeta), Mux3/2
  Sum3/1 -> 反Park/2(Q)
  Park/1(D) -> Mux/1, Sum2/2, 定子电流2/2  "id"
  Bus Selector/1 -> 电磁转矩Te/1, Tm/1  "<Electromagnetic torque Te (N*m)>"
  Bus Selector/5 -> Clark/2(B), Mux2/2  "<Stator current is_b (A)>"
  Bus Selector/2 -> Gain/1  "<Rotor angle thetam (rad)>"
  参考转速/1 -> Scope2/1, Sum5/1  "n"
  前馈解耦d轴补偿电压/1 -> Sum3/2
  ACR2/1 -> Sum3/1, 转速4/1
  Sum4/1 -> 反Park/1(D)
  SVPWM/1(pwm) -> Universal Bridge/1
  Mux1/1 -> 前馈解耦q轴补偿电压/1
  Gain2/1 -> Mux/2, Mux1/2  "we"
  Gain/1 -> Park/3(angle), 反Park/3(angle)
  Constant2/1 -> Sum2/1
  Bus Selector/4 -> Clark/3(C), Mux2/1  "<Stator current is_c (A)>"
  ACR1/1 -> Sum4/1, 转速3/1
  connections:
  Voltage Measurement/LConn1 -- Permanent Magnet Synchronous Machine1/LConn1 -- Universal Bridge/LConn1
  Voltage Measurement/LConn2 -- Permanent Magnet Synchronous Machine1/LConn2 -- Universal Bridge/LConn2
  DC/RConn1 -- Universal Bridge/RConn1
  Permanent Magnet Synchronous Machine1/LConn3 -- Universal Bridge/LConn3
  DC/LConn1 -- Universal Bridge/RConn2

== system MPC_FOC/负载 ==
  Demux : Demux  Tag=STV Demux  Outputs=3
      settings: DisplayOption=none
  FromWs : FromWorkspace  Tag=STV FromWs  VariableName=tuvar
      SigBuilderData=|
      | common.afterFinalStr = 'Extrapolate'
      | common.sampleTime = 0
      | dataSet.timeRange = [0 10]
      | dataSet.name = 'Group 1'
      | sbobj.Groups.Name = 'Group 1'
      | sbobj.Groups.Signals(1).Name = 'Signal 1'
      | sbobj.Groups.Signals(1).XData = [0 0.1 0.1 10]
      | sbobj.Groups.Signals(1).YData = [0 0.1 20 20]
      | sbobj.Groups.Signals(2).Name = 'Signal 2'
      | sbobj.Groups.Signals(2).XData = [0 0.8 0.8 1.2 1.2 10]
      | sbobj.Groups.Signals(2).YData = [10 10 50 50 10 10]
      | sbobj.Groups.Signals(3).Name = 'Signal 3'
      | sbobj.Groups.Signals(3).XData = [0 10]
      | sbobj.Groups.Signals(3).YData = [10 10]
  Signal 1 : Outport  Tag=STV Outport
  Signal 2 : Outport  Tag=STV Outport  Port=2
  Signal 3 : Outport  Tag=STV Outport  Port=3
  wires:
  Demux/3 -> Signal 3/1
  Demux/2 -> Signal 2/1
  Demux/1 -> Signal 1/1
  FromWs/1 -> Demux/1

== system MPC_FOC/负载1 ==
  Demux : Demux  Tag=STV Demux  Outputs=3
      settings: DisplayOption=none
  FromWs : FromWorkspace  Tag=STV FromWs  VariableName=tuvar
      SigBuilderData=|
      | common.afterFinalStr = 'Extrapolate'
      | common.sampleTime = 0
      | dataSet.timeRange = [0 10]
      | dataSet.name = 'Group 1'
      | sbobj.Groups.Name = 'Group 1'
      | sbobj.Groups.Signals(1).Name = 'Signal 1'
      | sbobj.Groups.Signals(1).XData = [0 0.1 0.1 10]
      | sbobj.Groups.Signals(1).YData = [0 0.1 20 20]
      | sbobj.Groups.Signals(2).Name = 'Signal 2'
      | sbobj.Groups.Signals(2).XData = [0 0.8 0.8 1.2 1.2 10]
      | sbobj.Groups.Signals(2).YData = [10 10 50 50 10 10]
      | sbobj.Groups.Signals(3).Name = 'Signal 3'
      | sbobj.Groups.Signals(3).XData = [0 10]
      | sbobj.Groups.Signals(3).YData = [10 10]
  Signal 1 : Outport  Tag=STV Outport
  Signal 2 : Outport  Tag=STV Outport  Port=2
  Signal 3 : Outport  Tag=STV Outport  Port=3
  wires:
  Demux/3 -> Signal 3/1
  Demux/2 -> Signal 2/1
  Demux/1 -> Signal 1/1
  FromWs/1 -> Demux/1

== system MPC_FOC/DVVMPC/Clark ==
  A : Inport
  B : Inport  Port=2
  C : Inport  Port=3
  Add : Sum
  Add1 : Sum  Inputs=+-
  Add2 : Sum  Inputs=+-
  Gain : Gain  Gain=0.5
  Gain1 : Gain  Gain=2/3
  Gain2 : Gain  Gain=1/sqrt(3)
  Alpha : Outport
  Beta : Outport  Port=2
  wires:
  B/1 -> Add2/1, Add/1
  C/1 -> Add/2, Add2/2
  Add/1 -> Gain/1
  A/1 -> Add1/1
  Gain/1 -> Add1/2
  Add1/1 -> Gain1/1
  Gain1/1 -> Alpha/1
  Add2/1 -> Gain2/1
  Gain2/1 -> Beta/1

== system MPC_FOC/DVVMPC/Park ==
  Alpha : Inport
  Beta : Inport  Port=2
  angle : Inport  Port=3
  Add1 : Sum
  Add2 : Sum  Inputs=-+
  Product{,1..3} (4 alike) : Product
  Trigonometric Function1 : Trigonometry
  Trigonometric Function2 : Trigonometry  Operator=cos
  D : Outport
  Q : Outport  Port=2
  wires:
  Add2/1 -> Q/1
  Product3/1 -> Add2/2
  Product2/1 -> Add2/1
  Add1/1 -> D/1
  Product1/1 -> Add1/2
  Product/1 -> Add1/1
  Trigonometric Function1/1 -> Product2/2, Product1/2
  Beta/1 -> Product3/1, Product1/1
  Trigonometric Function2/1 -> Product3/2, Product/2
  Alpha/1 -> Product2/1, Product/1
  angle/1 -> Trigonometric Function1/1, Trigonometric Function2/1

== system MPC_FOC/FOC/Clark ==
  A : Inport
  B : Inport  Port=2
  C : Inport  Port=3
  Add : Sum
  Add1 : Sum  Inputs=+-
  Add2 : Sum  Inputs=+-
  Gain : Gain  Gain=0.5
  Gain1 : Gain  Gain=2/3
  Gain2 : Gain  Gain=1/sqrt(3)
  Alpha : Outport
  Beta : Outport  Port=2
  wires:
  Gain2/1 -> Beta/1
  Add2/1 -> Gain2/1
  Gain1/1 -> Alpha/1
  Add1/1 -> Gain1/1
  Gain/1 -> Add1/2
  A/1 -> Add1/1
  Add/1 -> Gain/1
  C/1 -> Add2/2, Add/2
  B/1 -> Add/1, Add2/1

== system MPC_FOC/FOC/Park ==
  Alpha : Inport
  Beta : Inport  Port=2
  angle : Inport  Port=3
  Add1 : Sum
  Add2 : Sum  Inputs=-+
  Product{,1..3} (4 alike) : Product
  Trigonometric Function1 : Trigonometry
  Trigonometric Function2 : Trigonometry  Operator=cos
  D : Outport
  Q : Outport  Port=2
  wires:
  angle/1 -> Trigonometric Function2/1, Trigonometric Function1/1
  Alpha/1 -> Product/1, Product2/1
  Trigonometric Function2/1 -> Product/2, Product3/2
  Beta/1 -> Product1/1, Product3/1
  Trigonometric Function1/1 -> Product1/2, Product2/2
  Product/1 -> Add1/1
  Product1/1 -> Add1/2
  Add1/1 -> D/1
  Product2/1 -> Add2/1
  Product3/1 -> Add2/2
  Add2/1 -> Q/1

== system MPC_FOC/FOC/SVPWM ==
  Ualpha : Inport
  Ubeta : Inport  Port=2
  Constant : Constant  Value=0.0001
  Constant1 : Constant  Value=560
  PWM Generator : Subsystem
  Scope : Scope
  Scope1 : Scope
  Scope2 : Scope
  Sector Caculate : Subsystem
  T1T2 Caculate : Subsystem
  XYZ Caculate : Subsystem
  pwm : Outport
  wires:
  PWM Generator/1(pwm) -> Scope/1, pwm/1
  T1T2 Caculate/2(T2) -> PWM Generator/3(T2)
  T1T2 Caculate/1("T1 ") -> Scope2/1, PWM Generator/2(T1)
  Sector Caculate/1(N) -> PWM Generator/1(N), T1T2 Caculate/1(N), Scope1/1
  XYZ Caculate/1(XYZ) -> T1T2 Caculate/2(XYZ)
  Constant1/1 -> XYZ Caculate/4(Udc)
  Constant/1 -> XYZ Caculate/3(Ts), T1T2 Caculate/3(Tpwm), PWM Generator/4(T3)
  Ubeta/1 -> XYZ Caculate/2(Ubeta), Sector Caculate/2("Ubeta ")
  Ualpha/1 -> Sector Caculate/1(Ualpha), XYZ Caculate/1(Ualpha)

== system MPC_FOC/FOC/反Park ==
  D : Inport
  Q : Inport  Port=2
  angle : Inport  Port=3
  Add1 : Sum  Inputs=+-
  Add2 : Sum
  Product{,1..3} (4 alike) : Product
  Trigonometric Function1 : Trigonometry
  Trigonometric Function2 : Trigonometry  Operator=cos
  Alpha : Outport
  Beta : Outport  Port=2
  wires:
  Add2/1 -> Beta/1
  Product3/1 -> Add2/2
  Product2/1 -> Add2/1
  Add1/1 -> Alpha/1
  Product1/1 -> Add1/2
  Product/1 -> Add1/1
  Trigonometric Function1/1 -> Product2/2, Product1/2
  Q/1 -> Product3/1, Product1/1
  Trigonometric Function2/1 -> Product3/2, Product/2
  D/1 -> Product2/1, Product/1
  angle/1 -> Trigonometric Function1/1, Trigonometric Function2/1

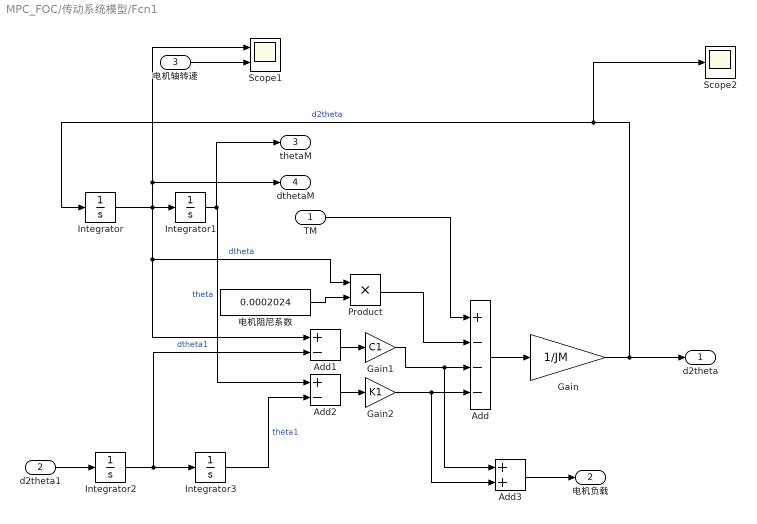
== system MPC_FOC/传动系统模型/Fcn1 ==
  TM : Inport
  d2theta1 : Inport  Port=2
  电机轴转速 : Inport  Port=3
  Add : Sum  Inputs=+---
  Add1 : Sum  Inputs=+-
  Add2 : Sum  Inputs=+-
  Add3 : Sum
  Gain : Gain  Gain=1/JM
  Gain1 : Gain  Gain=C1
  Gain2 : Gain  Gain=K1
  Integrator{,1..3} (4 alike) : Integrator
  Product : Product
  Scope1 : Scope  NumInputPorts=2
  Scope2 : Scope
  电机阻尼系数 : Constant  Value=0.0002024
  d2theta : Outport
  电机负载 : Outport  Port=2
  thetaM : Outport  Port=3
  dthetaM : Outport  Port=4
  wires:
  Integrator1/1 -> thetaM/1, Add2/1  "theta"
  Integrator2/1 -> Integrator3/1, Add1/2  "dtheta1"
  Integrator/1 -> Scope1/1, dthetaM/1, Product/1, Add1/1, Integrator1/1  "dtheta"
  Add/1 -> Gain/1
  Gain/1 -> Scope2/1, Integrator/1, d2theta/1  "d2theta"
  Add1/1 -> Gain1/1
  d2theta1/1 -> Integrator2/1
  Gain2/1 -> Add3/2, Add/4
  Add2/1 -> Gain2/1
  Integrator3/1 -> Add2/2  "theta1"
  Gain1/1 -> Add3/1, Add/3
  电机轴转速/1 -> Scope1/2
  电机阻尼系数/1 -> Product/2
  TM/1 -> Add/1
  Product/1 -> Add/2
  Add3/1 -> 电机负载/1

== system MPC_FOC/传动系统模型/Fcn2 ==
  TL : Inport
  d2thata : Inport  Port=2
  Add : Sum  Inputs=-++
  Add1 : Sum  Inputs=-+
  Add2 : Sum  Inputs=-+
  Gain : Gain  Gain=1/JL
  Gain1 : Gain  Gain=C1
  Gain2 : Gain  Gain=K1
  Integrator{,1..3} (4 alike) : Integrator
  Scope1 : Scope
  Scope2 : Scope
  d2thetaL : Outport
  thetaL : Outport  Port=2
  dthetaL : Outport  Port=3
  wires:
  Gain1/1 -> Add/2
  Integrator3/1 -> Add2/2  "theta"
  Add2/1 -> Gain2/1
  Gain2/1 -> Add/3
  Add1/1 -> Scope2/1, Gain1/1
  Gain/1 -> Integrator/1, d2thetaL/1  "d2theta1"
  Add/1 -> Gain/1
  Integrator/1 -> dthetaL/1, Add1/1, Integrator1/1  "dtheta1"
  Integrator2/1 -> Scope1/1, Add1/2, Integrator3/1  "dtheta"
  Integrator1/1 -> thetaL/1, Add2/1  "theta1"
  TL/1 -> Add/1
  d2thata/1 -> Integrator2/1

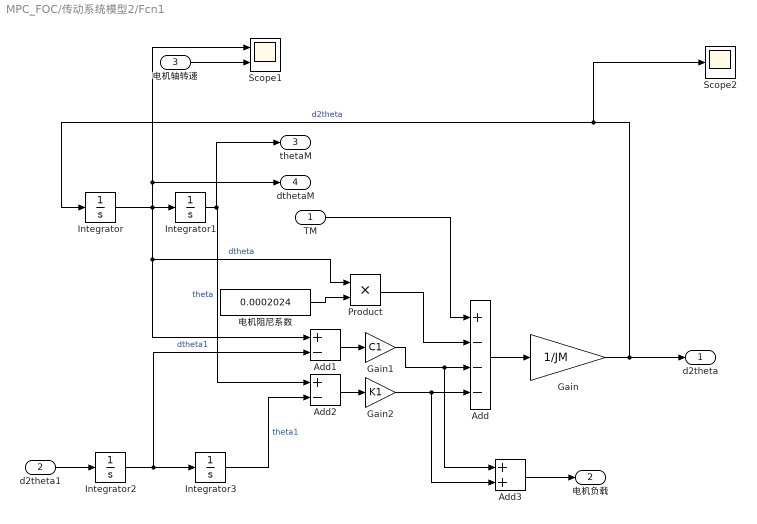
== system MPC_FOC/传动系统模型2/Fcn1 ==
  TM : Inport
  d2theta1 : Inport  Port=2
  电机轴转速 : Inport  Port=3
  Add : Sum  Inputs=+---
  Add1 : Sum  Inputs=+-
  Add2 : Sum  Inputs=+-
  Add3 : Sum
  Gain : Gain  Gain=1/JM
  Gain1 : Gain  Gain=C1
  Gain2 : Gain  Gain=K1
  Integrator{,1..3} (4 alike) : Integrator
  Product : Product
  Scope1 : Scope  NumInputPorts=2
  Scope2 : Scope
  电机阻尼系数 : Constant  Value=0.0002024
  d2theta : Outport
  电机负载 : Outport  Port=2
  thetaM : Outport  Port=3
  dthetaM : Outport  Port=4
  wires:
  Add3/1 -> 电机负载/1
  Product/1 -> Add/2
  TM/1 -> Add/1
  电机阻尼系数/1 -> Product/2
  电机轴转速/1 -> Scope1/2
  Gain1/1 -> Add/3, Add3/1
  Integrator3/1 -> Add2/2  "theta1"
  Add2/1 -> Gain2/1
  Gain2/1 -> Add/4, Add3/2
  d2theta1/1 -> Integrator2/1
  Add1/1 -> Gain1/1
  Gain/1 -> d2theta/1, Integrator/1, Scope2/1  "d2theta"
  Add/1 -> Gain/1
  Integrator/1 -> Integrator1/1, Add1/1, Product/1, dthetaM/1, Scope1/1  "dtheta"
  Integrator2/1 -> Add1/2, Integrator3/1  "dtheta1"
  Integrator1/1 -> Add2/1, thetaM/1  "theta"

== system MPC_FOC/传动系统模型2/Fcn2 ==
  TL : Inport
  d2thata : Inport  Port=2
  Add : Sum  Inputs=-++
  Add1 : Sum  Inputs=-+
  Add2 : Sum  Inputs=-+
  Gain : Gain  Gain=1/JL
  Gain1 : Gain  Gain=C1
  Gain2 : Gain  Gain=K1
  Integrator{,1..3} (4 alike) : Integrator
  Scope1 : Scope
  Scope2 : Scope
  d2thetaL : Outport
  thetaL : Outport  Port=2
  dthetaL : Outport  Port=3
  wires:
  d2thata/1 -> Integrator2/1
  TL/1 -> Add/1
  Integrator1/1 -> Add2/1, thetaL/1  "theta1"
  Integrator2/1 -> Integrator3/1, Add1/2, Scope1/1  "dtheta"
  Integrator/1 -> Integrator1/1, Add1/1, dthetaL/1  "dtheta1"
  Add/1 -> Gain/1
  Gain/1 -> d2thetaL/1, Integrator/1  "d2theta1"
  Add1/1 -> Gain1/1, Scope2/1
  Gain2/1 -> Add/3
  Add2/1 -> Gain2/1
  Integrator3/1 -> Add2/2  "theta"
  Gain1/1 -> Add/2

== system MPC_FOC/电机模型1/Clark ==
  A : Inport
  B : Inport  Port=2
  C : Inport  Port=3
  Add : Sum
  Add1 : Sum  Inputs=+-
  Add2 : Sum  Inputs=+-
  Gain : Gain  Gain=0.5
  Gain1 : Gain  Gain=2/3
  Gain2 : Gain  Gain=1/sqrt(3)
  Alpha : Outport
  Beta : Outport  Port=2
  wires:
  B/1 -> Add2/1, Add/1
  C/1 -> Add/2, Add2/2
  Add/1 -> Gain/1
  A/1 -> Add1/1
  Gain/1 -> Add1/2
  Add1/1 -> Gain1/1
  Gain1/1 -> Alpha/1
  Add2/1 -> Gain2/1
  Gain2/1 -> Beta/1

== system MPC_FOC/电机模型1/Park ==
  Alpha : Inport
  Beta : Inport  Port=2
  angle : Inport  Port=3
  Add1 : Sum
  Add2 : Sum  Inputs=-+
  Product{,1..3} (4 alike) : Product
  Trigonometric Function1 : Trigonometry
  Trigonometric Function2 : Trigonometry  Operator=cos
  D : Outport
  Q : Outport  Port=2
  wires:
  Add2/1 -> Q/1
  Product3/1 -> Add2/2
  Product2/1 -> Add2/1
  Add1/1 -> D/1
  Product1/1 -> Add1/2
  Product/1 -> Add1/1
  Trigonometric Function1/1 -> Product2/2, Product1/2
  Beta/1 -> Product3/1, Product1/1
  Trigonometric Function2/1 -> Product3/2, Product/2
  Alpha/1 -> Product2/1, Product/1
  angle/1 -> Trigonometric Function1/1, Trigonometric Function2/1

== system MPC_FOC/电机模型1/SVPWM ==
  Ualpha : Inport
  Ubeta : Inport  Port=2
  Constant : Constant  Value=0.0001
  Constant1 : Constant  Value=560
  PWM Generator : Subsystem
  Scope : Scope
  Scope1 : Scope
  Scope2 : Scope
  Sector Caculate : Subsystem
  T1T2 Caculate : Subsystem
  XYZ Caculate : Subsystem
  pwm : Outport
  wires:
  Ualpha/1 -> XYZ Caculate/1(Ualpha), Sector Caculate/1(Ualpha)
  Ubeta/1 -> Sector Caculate/2("Ubeta "), XYZ Caculate/2(Ubeta)
  Constant/1 -> PWM Generator/4(T3), T1T2 Caculate/3(Tpwm), XYZ Caculate/3(Ts)
  Constant1/1 -> XYZ Caculate/4(Udc)
  XYZ Caculate/1(XYZ) -> T1T2 Caculate/2(XYZ)
  Sector Caculate/1(N) -> Scope1/1, T1T2 Caculate/1(N), PWM Generator/1(N)
  T1T2 Caculate/1("T1 ") -> PWM Generator/2(T1), Scope2/1
  T1T2 Caculate/2(T2) -> PWM Generator/3(T2)
  PWM Generator/1(pwm) -> pwm/1, Scope/1

== system MPC_FOC/电机模型1/反Park ==
  D : Inport
  Q : Inport  Port=2
  angle : Inport  Port=3
  Add1 : Sum  Inputs=+-
  Add2 : Sum
  Product{,1..3} (4 alike) : Product
  Trigonometric Function1 : Trigonometry
  Trigonometric Function2 : Trigonometry  Operator=cos
  Alpha : Outport
  Beta : Outport  Port=2
  wires:
  angle/1 -> Trigonometric Function2/1, Trigonometric Function1/1
  D/1 -> Product/1, Product2/1
  Trigonometric Function2/1 -> Product/2, Product3/2
  Q/1 -> Product1/1, Product3/1
  Trigonometric Function1/1 -> Product1/2, Product2/2
  Product/1 -> Add1/1
  Product1/1 -> Add1/2
  Add1/1 -> Alpha/1
  Product2/1 -> Add2/1
  Product3/1 -> Add2/2
  Add2/1 -> Beta/1

== system MPC_FOC/电机模型2/Clark ==
  A : Inport
  B : Inport  Port=2
  C : Inport  Port=3
  Add : Sum
  Add1 : Sum  Inputs=+-
  Add2 : Sum  Inputs=+-
  Gain : Gain  Gain=0.5
  Gain1 : Gain  Gain=2/3
  Gain2 : Gain  Gain=1/sqrt(3)
  Alpha : Outport
  Beta : Outport  Port=2
  wires:
  Gain2/1 -> Beta/1
  Add2/1 -> Gain2/1
  Gain1/1 -> Alpha/1
  Add1/1 -> Gain1/1
  Gain/1 -> Add1/2
  A/1 -> Add1/1
  Add/1 -> Gain/1
  C/1 -> Add2/2, Add/2
  B/1 -> Add/1, Add2/1

== system MPC_FOC/电机模型2/Park ==
  Alpha : Inport
  Beta : Inport  Port=2
  angle : Inport  Port=3
  Add1 : Sum
  Add2 : Sum  Inputs=-+
  Product{,1..3} (4 alike) : Product
  Trigonometric Function1 : Trigonometry
  Trigonometric Function2 : Trigonometry  Operator=cos
  D : Outport
  Q : Outport  Port=2
  wires:
  angle/1 -> Trigonometric Function2/1, Trigonometric Function1/1
  Alpha/1 -> Product/1, Product2/1
  Trigonometric Function2/1 -> Product/2, Product3/2
  Beta/1 -> Product1/1, Product3/1
  Trigonometric Function1/1 -> Product1/2, Product2/2
  Product/1 -> Add1/1
  Product1/1 -> Add1/2
  Add1/1 -> D/1
  Product2/1 -> Add2/1
  Product3/1 -> Add2/2
  Add2/1 -> Q/1

== system MPC_FOC/电机模型2/SVPWM ==
  Ualpha : Inport
  Ubeta : Inport  Port=2
  Constant : Constant  Value=0.0001
  Constant1 : Constant  Value=560
  PWM Generator : Subsystem
  Scope : Scope
  Scope1 : Scope
  Scope2 : Scope
  Sector Caculate : Subsystem
  T1T2 Caculate : Subsystem
  XYZ Caculate : Subsystem
  pwm : Outport
  wires:
  PWM Generator/1(pwm) -> Scope/1, pwm/1
  T1T2 Caculate/2(T2) -> PWM Generator/3(T2)
  T1T2 Caculate/1("T1 ") -> Scope2/1, PWM Generator/2(T1)
  Sector Caculate/1(N) -> PWM Generator/1(N), T1T2 Caculate/1(N), Scope1/1
  XYZ Caculate/1(XYZ) -> T1T2 Caculate/2(XYZ)
  Constant1/1 -> XYZ Caculate/4(Udc)
  Constant/1 -> XYZ Caculate/3(Ts), T1T2 Caculate/3(Tpwm), PWM Generator/4(T3)
  Ubeta/1 -> XYZ Caculate/2(Ubeta), Sector Caculate/2("Ubeta ")
  Ualpha/1 -> Sector Caculate/1(Ualpha), XYZ Caculate/1(Ualpha)

== system MPC_FOC/电机模型2/反Park ==
  D : Inport
  Q : Inport  Port=2
  angle : Inport  Port=3
  Add1 : Sum  Inputs=+-
  Add2 : Sum
  Product{,1..3} (4 alike) : Product
  Trigonometric Function1 : Trigonometry
  Trigonometric Function2 : Trigonometry  Operator=cos
  Alpha : Outport
  Beta : Outport  Port=2
  wires:
  Add2/1 -> Beta/1
  Product3/1 -> Add2/2
  Product2/1 -> Add2/1
  Add1/1 -> Alpha/1
  Product1/1 -> Add1/2
  Product/1 -> Add1/1
  Trigonometric Function1/1 -> Product2/2, Product1/2
  Q/1 -> Product3/1, Product1/1
  Trigonometric Function2/1 -> Product3/2, Product/2
  D/1 -> Product2/1, Product/1
  angle/1 -> Trigonometric Function1/1, Trigonometric Function2/1

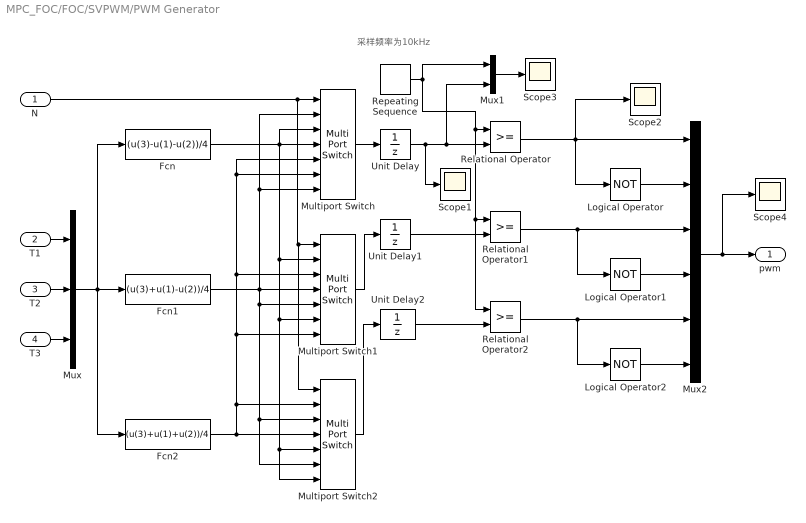
== system MPC_FOC/FOC/SVPWM/PWM Generator ==
  note: 采样频率为10kHz
  N : Inport
  T1 : Inport  Port=2
  T2 : Inport  Port=3
  T3 : Inport  Port=4
  Fcn : Fcn  Expr=(u(3)-u(1)-u(2))/4
  Fcn1 : Fcn  Expr=(u(3)+u(1)-u(2))/4
  Fcn2 : Fcn  Expr=(u(3)+u(1)+u(2))/4
  Logical Operator : Logic  Operator=NOT  AllPortsSameDT=off  OutDataTypeStr=boolean
  Logical Operator1 : Logic  Operator=NOT  AllPortsSameDT=off  OutDataTypeStr=boolean
  Logical Operator2 : Logic  Operator=NOT  AllPortsSameDT=off  OutDataTypeStr=boolean
  Multiport Switch : MultiPortSwitch  Inputs=6  DiagnosticForDefault=None
  Multiport Switch1 : MultiPortSwitch  Inputs=6  DiagnosticForDefault=None
  Multiport Switch2 : MultiPortSwitch  Inputs=6  DiagnosticForDefault=None
  Mux : Mux  Inputs=3
  Mux1 : Mux  Inputs=2
  Mux2 : Mux  Inputs=6
  Relational Operator : RelationalOperator  OutDataTypeStr=boolean  RndMeth=Nearest
  Relational Operator1 : RelationalOperator  OutDataTypeStr=boolean  RndMeth=Nearest
  Relational Operator2 : RelationalOperator  OutDataTypeStr=boolean  RndMeth=Nearest
  Repeating Sequence : simulink/Sources/Repeating Sequence  rep_seq_t=[0 0.00005 0.0001]  rep_seq_y=[0 0.00005 0]
  Scope{1..4} (4 alike) : Scope
  Unit Delay : UnitDelay  SampleTime=0.0001  HasFrameUpgradeWarning=on
  Unit Delay1 : UnitDelay  SampleTime=0.0001  HasFrameUpgradeWarning=on
  Unit Delay2 : UnitDelay  SampleTime=0.0001  HasFrameUpgradeWarning=on
  pwm : Outport
  wires:
  Unit Delay2/1 -> Relational Operator2/2
  Unit Delay1/1 -> Relational Operator1/2
  Unit Delay/1 -> Scope1/1, Relational Operator/2, Mux1/2
  Mux1/1 -> Scope3/1
  Multiport Switch/1 -> Unit Delay/1
  Multiport Switch2/1 -> Unit Delay2/1
  Multiport Switch1/1 -> Unit Delay1/1
  Mux2/1 -> pwm/1, Scope4/1
  Logical Operator2/1 -> Mux2/6
  Logical Operator1/1 -> Mux2/4
  Logical Operator/1 -> Mux2/2
  Relational Operator2/1 -> Mux2/5, Logical Operator2/1
  Relational Operator1/1 -> Mux2/3, Logical Operator1/1
  Relational Operator/1 -> Mux2/1, Logical Operator/1, Scope2/1
  Repeating Sequence/1 -> Relational Operator/1, Relational Operator1/1, Relational Operator2/1, Mux1/1
  Fcn2/1 -> Multiport Switch/5, Multiport Switch/6, Multiport Switch1/3, Multiport Switch1/7, Multiport Switch2/2, Multiport Switch2/4
  Fcn1/1 -> Multiport Switch1/4, Multiport Switch1/5, Multiport Switch2/3, Multiport Switch2/6, Multiport Switch/2, Multiport Switch/7
  Fcn/1 -> Multiport Switch/3, Multiport Switch/4, Multiport Switch1/2, Multiport Switch1/6, Multiport Switch2/5, Multiport Switch2/7
  N/1 -> Multiport Switch/1, Multiport Switch1/1, Multiport Switch2/1
  Mux/1 -> Fcn2/1, Fcn1/1, Fcn/1
  T3/1 -> Mux/3
  T1/1 -> Mux/1
  T2/1 -> Mux/2

== system MPC_FOC/FOC/SVPWM/Sector Caculate ==
  Ualpha : Inport
  "Ubeta " : Inport  Port=2
  Add : Sum  Inputs=+++
  Add1 : Sum  Inputs=+-
  Add2 : Sum  Inputs=--
  Constant : Constant
  Constant1 : Constant  Value=0
  Constant2 : Constant  Value=3/4
  Gain : Gain  Gain=4
  Gain1 : Gain  Gain=2
  Gain2 : Gain  Gain=0.5
  Product : Product
  Sqrt : Sqrt  SaturateOnIntegerOverflow=on
  Switch : Switch  Criteria=u2 > Threshold
  Switch1 : Switch  Criteria=u2 > Threshold
  Switch2 : Switch  Criteria=u2 > Threshold
  N : Outport
  wires:
  Gain2/1 -> Add2/2, Add1/2
  Product/1 -> Add1/1, Add2/1
  Sqrt/1 -> Product/2
  Constant2/1 -> Sqrt/1
  Switch/1 -> Add/1
  Switch1/1 -> Gain1/1
  Switch2/1 -> Gain/1
  Gain/1 -> Add/3
  Gain1/1 -> Add/2
  Add/1 -> N/1
  Constant1/1 -> Switch/3, Switch1/3, Switch2/3
  Constant/1 -> Switch2/1, Switch1/1, Switch/1
  Add2/1 -> Switch2/2
  Add1/1 -> Switch1/2
  "Ubeta "/1 -> Gain2/1, Switch/2
  Ualpha/1 -> Product/1

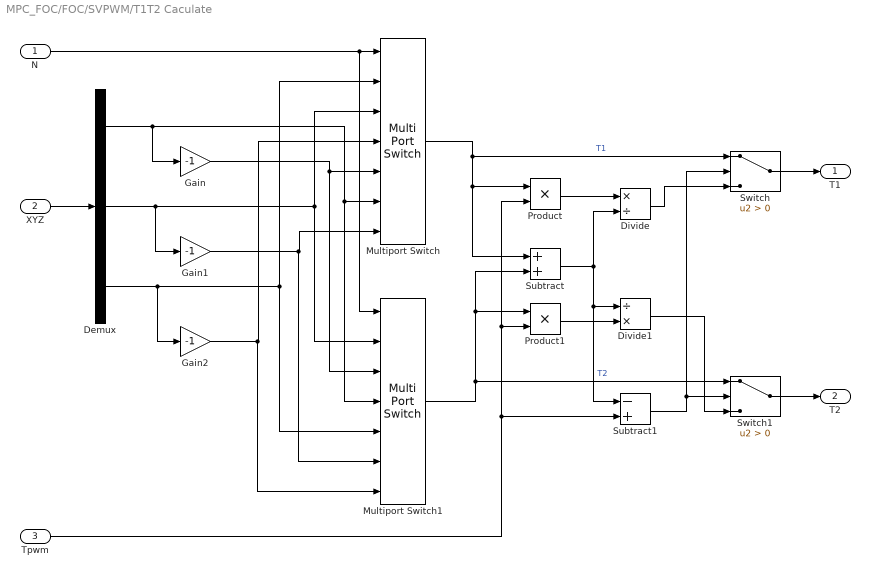
== system MPC_FOC/FOC/SVPWM/T1T2 Caculate ==
  N : Inport
  XYZ : Inport  Port=2
  Tpwm : Inport  Port=3
  Demux : Demux  Outputs=3
  Divide : Product  Inputs=*/
  Divide1 : Product  Inputs=/*
  Gain : Gain  Gain=-1
  Gain1 : Gain  Gain=-1
  Gain2 : Gain  Gain=-1
  Multiport Switch : MultiPortSwitch  Inputs=6  DiagnosticForDefault=None
  Multiport Switch1 : MultiPortSwitch  Inputs=6  DiagnosticForDefault=None
  Product : Product
  Product1 : Product
  Subtract : Sum
  Subtract1 : Sum  Inputs=-+
  Switch : Switch  Criteria=u2 > Threshold
  Switch1 : Switch  Criteria=u2 > Threshold
  "T1 " : Outport
  T2 : Outport  Port=2
  wires:
  Product1/1 -> Divide1/2
  Subtract/1 -> Subtract1/1, Divide1/1, Divide/2
  Product/1 -> Divide/1
  Switch/1 -> "T1 "/1
  Switch1/1 -> T2/1
  Subtract1/1 -> Switch/2, Switch1/2
  Divide1/1 -> Switch1/3
  Divide/1 -> Switch/3
  Tpwm/1 -> Product1/2, Product/2, Subtract1/2
  Multiport Switch1/1 -> Switch1/1, Product1/1, Subtract/2  "T2"
  Multiport Switch/1 -> Subtract/1, Product/1, Switch/1  "T1"
  XYZ/1 -> Demux/1
  Gain2/1 -> Multiport Switch/4, Multiport Switch1/7
  Gain1/1 -> Multiport Switch/7, Multiport Switch1/6
  Gain/1 -> Multiport Switch1/3, Multiport Switch/5
  Demux/3 -> Multiport Switch/2, Multiport Switch1/5, Gain2/1
  Demux/2 -> Gain1/1, Multiport Switch1/2, Multiport Switch/3
  Demux/1 -> Gain/1, Multiport Switch/6, Multiport Switch1/4
  N/1 -> Multiport Switch/1, Multiport Switch1/1
